simulink model "control_model_5"  (R2025b)
settings: Solver=VariableStepAuto  StartTime=0.0  StopTime=500  RelTol=1e-3
values from neighbouring files (symbols this model uses):
  Am = [0 1 0 0; -walpha^2 -2*zeta_alpha*walpha 0 0; 0 0 0 1; 0 0 -wgamma^2 -2*zeta_gamma*wgamma]    [main_v2.m]    (also in script_plane.m = [0 1; -wn^2 -2*zeta*wn])
  B = [0; Cm_delta*K/Iy; 0; 0]    [main_v2.m]    (also in script_plane.m = [0; Cm_delta/Iy])
  Bm = [0; walpha^2; 0; 0]    [main_v2.m]    (also in script_plane.m = [0; wn^2])
  c = 3.2    [main_v2.m]    (also in script_plane.m = 3.45)
  Cd0 = 0.02    [main_v2.m]
  Cl0 = 0.1    [main_v2.m]
  Cl_alpha = 5.7    [main_v2.m]
  Cm_0 = -0.8    [main_v2.m]
  Cm_delta = -0.5    [main_v2.m]    (also in script_plane.m = -1)
  Cm_q = -12    [main_v2.m]    (also in script_plane.m = -8)
  delta_max = deg2rad(25)    [main_v2.m]    (also in script_plane.m)
  desired_aoa = deg2rad(45)    [main_v2.m]    (also in script_plane.m = deg2rad(20))
  g = 9.81    [main_v2.m]
  gain_e = 0.1    [main_v2.m]    (also in script_plane.m = 50000)
  gain_r = 0.01    [main_v2.m]    (also in script_plane.m = 500000)
  gain_x = 0.00002    (= 2e-05)    [main_v2.m]    (also in script_plane.m = 500000)
  Iy = 160000    [main_v2.m]    (also in script_plane.m = 70000)
  K = 1/2 *rho * S *c    (= 58.8)    [main_v2.m]    (also in script_plane.m = 1908126.5175)
  k_d1 = 0.045    [main_v2.m]
  k_d2 = 0.08    [main_v2.m]
  kl = 3    [main_v2.m]
  Kr = 34.3*10^-3    (= 0.0343)    [main_v2.m]    (also in script_plane.m = -0.825)
  Kx = [19 -8 0 15]*10^-5    [main_v2.m]    (also in script_plane.m = [1.33 0.15])
  mass = 9000    [main_v2.m]    (also in script_plane.m = 12000)
  P = lyap(Am',Q)    [main_v2.m]    (also in script_plane.m)
  rate_of_change = 4    [main_v2.m]    (also in script_plane.m = 15)
  rate_of_freeze_angle = 1    [main_v2.m]
  rate_of_freeze_rate = 2    [main_v2.m]
  rho = 1.225    [main_v2.m]    (also in script_plane.m)
  S = 30    [main_v2.m]    (also in script_plane.m = 27.87)
  sigma_r = 0.001    [main_v2.m]    (also in script_plane.m = 0.0002)
  sigma_w = 0.001    [main_v2.m]    (also in script_plane.m = 0.0002)
  sigma_x = 0.001    [main_v2.m]    (also in script_plane.m = 0.0002)
  speed = 180    [main_v2.m]    (also in script_plane.m)
  thrust = 160000    [main_v2.m]
  W = [0 0 0 0 0]*10^-6    [main_v2.m]    (also in script_plane.m = [0 0 0 0])
  zeta_alpha = 1    [main_v2.m]
libraries: simulink_extras x22, simulink x2, slctrl_adaptive x1
settings Model: Creator=marti  LastModifiedBy=marti
settings SolverCC: ZeroCrossAlgorithm=Adaptive
settings DebuggingCC: MaskedZcDiagnostic=none  IgnoredZcDiagnostic=none

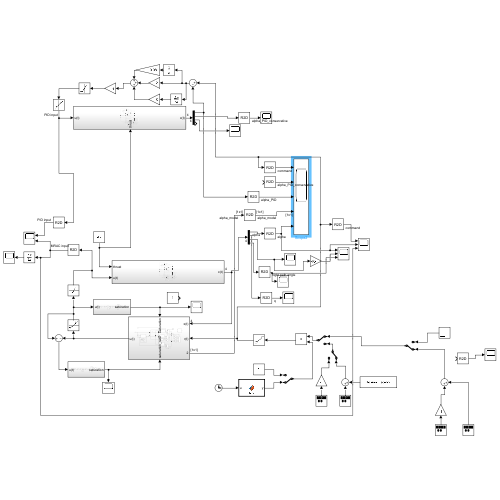
[thumbnail: Simulink's stored preview of the top-level diagram]
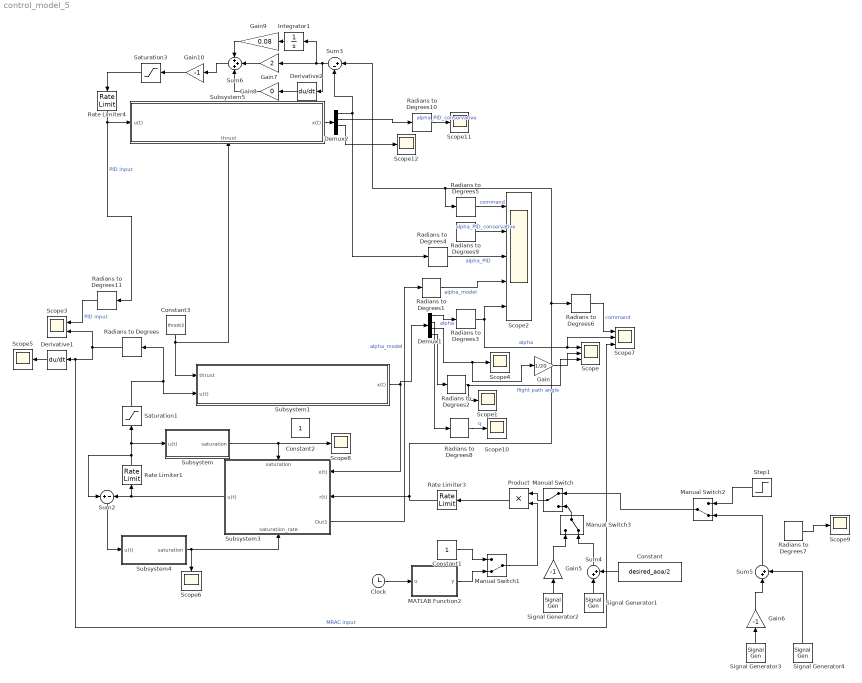
== system control_model_5 ==
  Clock : Clock
  Constant : Constant  Value=desired_aoa/2
  Constant1 : Constant
  Constant2 : Constant
  Constant3 : Constant  Value=thrust/3
  Demux1 : Demux
  Demux2 : Demux
  Derivative1 : Derivative
  Derivative2 : Derivative
  Gain : Gain  Gain=1/20
  Gain10 : Gain  Gain=-1
  Gain5 : Gain  Gain=-1
  Gain6 : Gain  Gain=-1
  Gain7 : Gain  Gain=2
  Gain8 : Gain  Gain=0
  Gain9 : Gain  Gain=0.08
  Integrator1 : Integrator
  MATLAB Function2 : MATLAB Function  TreatAsAtomicUnit=on
  Manual Switch : ManualSwitch
  Manual Switch1 : ManualSwitch  CurrentSetting=0
  Manual Switch2 : ManualSwitch  CurrentSetting=0
  Manual Switch3 : ManualSwitch  CurrentSetting=0
  Product : Product
  Radians to Degrees{,1..11} (12 alike) : simulink_extras/Transformations/Radians to Degrees
  Rate Limiter1 : RateLimiter  RisingSlewLimit=deg2rad(60)  FallingSlewLimit=-deg2rad(60)  SampleTimeMode=inherited
  Rate Limiter3 : RateLimiter  RisingSlewLimit=deg2rad(50)  FallingSlewLimit=-deg2rad(50)  SampleTimeMode=inherited
  Rate Limiter4 : RateLimiter  RisingSlewLimit=deg2rad(60)  FallingSlewLimit=-deg2rad(60)  SampleTimeMode=inherited
  Saturation1 : Saturate  UpperLimit=delta_max  LowerLimit=-delta_max  ZeroCross=off
  Saturation3 : Saturate  UpperLimit=delta_max  LowerLimit=-delta_max  ZeroCross=off
  Scope : Scope  NumInputPorts=3
      settings: ActiveDisplayYMinimum=-1  ActiveDisplayYMaximum=1  DataLoggingVariableName=ScopeData3
  Scope{1,4..6,8..12} (9 alike) : Scope
      Scope1 settings: ActiveDisplayYMinimum=-58.129213057968116  ActiveDisplayYMaximum=60.751359776371949  DataLoggingVariableName=ScopeData2
      Scope10 settings: ActiveDisplayYMinimum=-62.75251155469028  ActiveDisplayYMaximum=72.596643379359037  DataLoggingVariableName=ScopeData21
      Scope11 settings: ActiveDisplayYMinimum=-64.708088733273414  ActiveDisplayYMaximum=63.8671469407195  DataLoggingVariableName=ScopeData25
      Scope12 settings: ActiveDisplayYMinimum=129.65199773274497  ActiveDisplayYMaximum=311.01554736607403  DataLoggingVariableName=ScopeData26
      Scope4 settings: ActiveDisplayYMinimum=70.6671051217048  ActiveDisplayYMaximum=318.87721463336675  DataLoggingVariableName=ScopeData13
      Scope5 settings: ActiveDisplayYMinimum=-75.0023145799513  ActiveDisplayYMaximum=75.004597453327918  DataLoggingVariableName=ScopeData17
      Scope6 settings: ActiveDisplayYMinimum=-0.12499999999999997  ActiveDisplayYMaximum=1.125  DataLoggingVariableName=ScopeData12
      Scope8 settings: ActiveDisplayYMinimum=0.14902753825083676  ActiveDisplayYMaximum=1.0945524934597364  DataLoggingVariableName=ScopeData18
      Scope9 settings: ActiveDisplayYMinimum=-1  ActiveDisplayYMaximum=1  DataLoggingVariableName=ScopeData19
  Scope2 : Scope  NumInputPorts=5
      settings: ActiveDisplayYMinimum=-57.336392914968393  ActiveDisplayYMaximum=57.316790282004284  DataLoggingVariableName=ScopeData15
  Scope3 : Scope  NumInputPorts=2
      settings: ActiveDisplayYMinimum=-26.434953423968707  ActiveDisplayYMaximum=30.698276071875242  DataLoggingVariableName=ScopeData16
  Scope7 : Scope  NumInputPorts=3
      settings: ActiveDisplayYMinimum=-76.904040190876856  ActiveDisplayYMaximum=77.107808461045764  DataLoggingVariableName=ScopeData14
  Signal Generator1 : SignalGenerator  WaveForm=square  Amplitude=desired_aoa/2  Frequency=0.1  Units=rad/sec
  Signal Generator2 : SignalGenerator  WaveForm=square  Amplitude=desired_aoa  Frequency=0.2  Units=rad/sec
  Signal Generator3 : SignalGenerator  WaveForm=square  Amplitude=desired_aoa/2  Frequency=0.1  Units=rad/sec
  Signal Generator4 : SignalGenerator  WaveForm=square  Amplitude=desired_aoa/2  Frequency=0.05  Units=rad/sec
  Step1 : Step  Time=31.3  After=desired_aoa  SampleTime=0
  Subsystem : Subsystem
  Subsystem1 : Subsystem
  Subsystem3 : Subsystem
      settings: PortSchema="{\"entries\":[{\"content\":{\"sides\":[{\"content\":{\"connectorIds\":[\"Out2\",\"In1\",\"In2\"]},\"type\":\"ConnectorPlacement.EquallySpacedRectSide\",\"uuid\":\"2a5405b8-f474-466f-9064-f86b75893dd0\"},{\"content\":{\"connectorIds\":[\"Out1\"],\"side\":\"RIGHT\"},\"type\":\"ConnectorPlacement.EquallySpacedRectSide\",\"uuid\":\"ad673661-f4e9-494b-83cc-7452eec3fe31\"},{\"content\":{\"connectorIds\":[\"In3\"],\"side\":\"TOP\"},\"type\":\"ConnectorPlacement.EquallySpacedRectSide\",\"uuid\":\"21a76317-3288-4ff3-bd02-68708e86e3a8\"},{\"content\":{\"connectorIds\":[\"In4\"],\"side\":\"BOTTOM\"},\"type\":\"ConnectorPlacement.EquallySpacedRectSide\",\"uuid\":\"06318006-2373-43e5-8136-a784e8462fed\"}]},\"type\":\"ConnectorPlacement.EquallySpacedConnector\",\"uuid\":\"fc0ce599-928f-4c66-9629-0b98f2391e21\"}],\"packageUris\":[\"http://schema.mathworks.com/mf0/Connector/R2020b\"],\"version\":\"1.0\"}"
  Subsystem4 : Subsystem
  Subsystem5 : Subsystem
      settings: PortSchema="{\"entries\":[{\"content\":{\"sides\":[{\"content\":{\"connectorIds\":[\"In1\"]},\"type\":\"ConnectorPlacement.EquallySpacedRectSide\",\"uuid\":\"e785faf8-3185-4a85-a8dc-ea057f593b7d\"},{\"content\":{\"connectorIds\":[\"Out1\"],\"side\":\"RIGHT\"},\"type\":\"ConnectorPlacement.EquallySpacedRectSide\",\"uuid\":\"50c2acdd-3993-4760-8234-c723508cab38\"},{\"content\":{\"side\":\"TOP\"},\"type\":\"ConnectorPlacement.EquallySpacedRectSide\",\"uuid\":\"23fa212d-a38a-4506-9cd4-8e0f9463f517\"},{\"content\":{\"connectorIds\":[\"In2\"],\"side\":\"BOTTOM\"},\"type\":\"ConnectorPlacement.EquallySpacedRectSide\",\"uuid\":\"8bce308f-c5df-4db2-bea6-6d2a873f00b4\"}]},\"type\":\"ConnectorPlacement.EquallySpacedConnector\",\"uuid\":\"334871f8-06ef-498c-97e4-8f1bab52b431\"}],\"packageUris\":[\"http://schema.mathworks.com/mf0/Connector/R2020b\"],\"version\":\"1.0\"}"
  Sum2 : Sum  Inputs=+|-
  Sum3 : Sum  Inputs=|+-
  Sum4 : Sum  Inputs=|++
  Sum5 : Sum  Inputs=|++
  Sum6 : Sum  Inputs=+++
  wires:
  Radians to Degrees3/1 -> Scope7/2, Scope/1, Scope2/5  "alpha"
  Radians to Degrees4/1 -> Scope2/3  "alpha_PID"
  Signal Generator1/1 -> Sum4/1
  Derivative1/1 -> Scope5/1
  Subsystem3/1(u(t)) -> Sum2/2, Rate Limiter1/1
  Subsystem4/1(saturation) -> Subsystem3/3(saturation_rate), Scope6/1
  Subsystem3/2(Out1) -> Radians to Degrees1/1  "alpha_model"
  Saturation1/1 -> Radians to Degrees/1, Subsystem1/2(u(t))
  Radians to Degrees1/1 -> Scope2/4  "alpha_model"
  Constant/1 -> Sum4/2
  Manual Switch3/1 -> Manual Switch/2
  Sum2/1 -> Subsystem4/1(u(t))
  Radians to Degrees5/1 -> Scope2/1  "command"
  Radians to Degrees/1 -> Scope3/2, Scope7/3, Derivative1/1  "MRAC input"
  Sum4/1 -> Manual Switch3/2
  Demux1/3 -> Gain/1, Scope4/1
  Radians to Degrees2/1 -> Scope1/1, Scope/3  "flight path angle"
  Clock/1 -> MATLAB Function2/1(u)
  Manual Switch/1 -> Product/1
  Demux1/1 -> Radians to Degrees3/1  "alpha"
  Demux1/4 -> Radians to Degrees2/1
  Constant1/1 -> Manual Switch1/1
  MATLAB Function2/1(y) -> Manual Switch1/2
  Manual Switch1/1 -> Product/2
  Gain/1 -> Scope/2
  Subsystem/1(saturation) -> Scope8/1, Subsystem3/4(saturation)
  Rate Limiter1/1 -> Sum2/1, Saturation1/1, Subsystem/1(u(t))
  Signal Generator2/1 -> Gain5/1
  Gain5/1 -> Manual Switch3/1
  Radians to Degrees6/1 -> Scope7/1  "command"
  Subsystem1/1(x(t)) -> Demux1/1, Subsystem3/2(x(t))
  Constant3/1 -> Subsystem5/2(thrust), Subsystem1/1(thrust)
  Signal Generator3/1 -> Gain6/1
  Gain6/1 -> Sum5/1
  Signal Generator4/1 -> Sum5/2
  Radians to Degrees7/1 -> Scope9/1
  Radians to Degrees8/1 -> Scope10/1  "q"
  Demux1/2 -> Radians to Degrees8/1
  Subsystem5/1(x(t)) -> Demux2/1
  Gain8/1 -> Sum6/3
  Gain9/1 -> Sum6/1
  Sum3/1 -> Derivative2/1, Gain7/1, Integrator1/1
  Derivative2/1 -> Gain8/1
  Gain10/1 -> Saturation3/1
  Demux2/1 -> Radians to Degrees4/1, Sum3/2
  Rate Limiter4/1 -> Radians to Degrees11/1, Subsystem5/1(u(t))  "PID input"
  Sum6/1 -> Gain10/1
  Rate Limiter3/1 -> Subsystem3/1(r(t)), Radians to Degrees5/1, Sum3/1, Radians to Degrees6/1
  Saturation3/1 -> Rate Limiter4/1
  Gain7/1 -> Sum6/2
  Radians to Degrees9/1 -> Scope2/2  "alpha_PID_conservative"
  Integrator1/1 -> Gain9/1
  Demux2/2 -> Radians to Degrees10/1
  Radians to Degrees10/1 -> Scope11/1  "alpha_PID_conservative"
  Demux2/3 -> Scope12/1
  Radians to Degrees11/1 -> Scope3/1  "PID input"
  Product/1 -> Rate Limiter3/1
  Manual Switch2/1 -> Manual Switch/1
  Sum5/1 -> Manual Switch2/2
  Step1/1 -> Manual Switch2/1

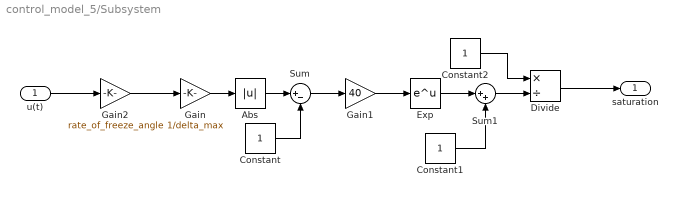
== system control_model_5/Subsystem ==
  u(t) : Inport
  Abs : Abs  SaturateOnIntegerOverflow=off
  Constant : Constant
  Constant1 : Constant
  Constant2 : Constant
  Divide : Product  Inputs=*/
  Exp : Math
  Gain : Gain  Gain=1/delta_max
  Gain1 : Gain  Gain=40
  Gain2 : Gain  Gain=rate_of_freeze_angle
  Sum : Sum  Inputs=|+-
  Sum1 : Sum  Inputs=|++
  saturation : Outport
  wires:
  Gain/1 -> Abs/1
  Abs/1 -> Sum/1
  Sum/1 -> Gain1/1
  Constant/1 -> Sum/2
  Gain1/1 -> Exp/1
  Exp/1 -> Sum1/1
  Constant1/1 -> Sum1/2
  Sum1/1 -> Divide/2
  Constant2/1 -> Divide/1
  Divide/1 -> saturation/1
  Gain2/1 -> Gain/1
  u(t)/1 -> Gain2/1

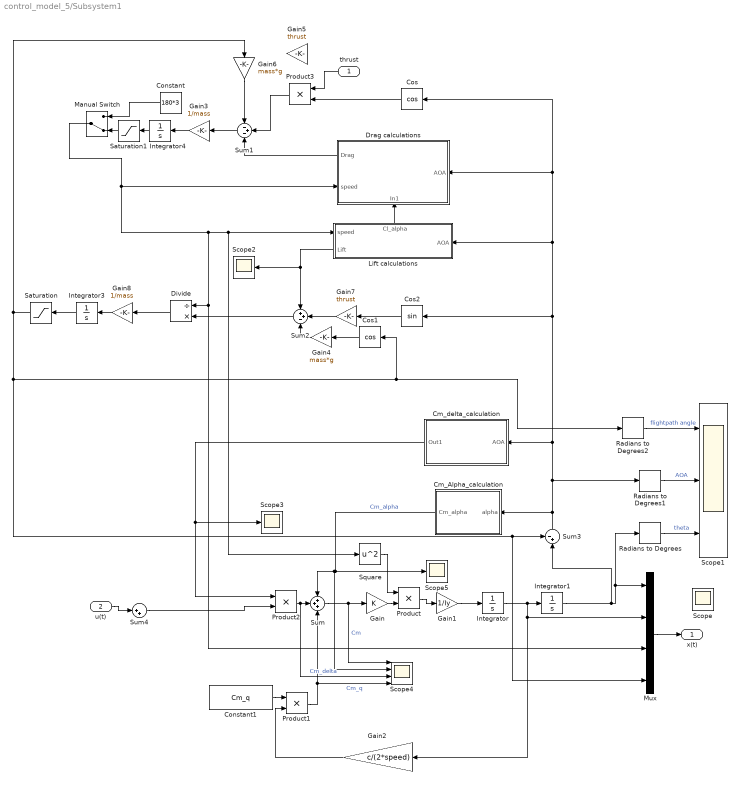
== system control_model_5/Subsystem1 ==
  thrust : Inport
  u(t) : Inport  Port=2
  Cm_Alpha_calculation : Subsystem
  Cm_delta_calculation : Subsystem
  Constant : Constant  Value=180*3
  Constant1 : Constant  Value=Cm_q
  Cos : Trigonometry  Operator=cos
  Cos1 : Trigonometry  Operator=cos
  Cos2 : Trigonometry
  Divide : Product  Inputs=/*
  Drag calculations : Subsystem
      settings: PortSchema="{\"entries\":[{\"content\":{\"sides\":[{\"content\":{\"connectorIds\":[\"Out1\",\"In1\"]},\"type\":\"ConnectorPlacement.EquallySpacedRectSide\",\"uuid\":\"d271dd9c-4b6b-493d-a484-ea343b2a7ea5\"},{\"content\":{\"connectorIds\":[\"In3\"],\"side\":\"RIGHT\"},\"type\":\"ConnectorPlacement.EquallySpacedRectSide\",\"uuid\":\"1c3a3b91-ae49-4f86-b72d-44481f1c47ea\"},{\"content\":{\"side\":\"TOP\"},\"type\":\"ConnectorPlacement.EquallySpacedRectSide\",\"uuid\":\"ad2c4e7a-6e16-439a-a8ce-91c789fc2dda\"},{\"content\":{\"connectorIds\":[\"In2\"],\"side\":\"BOTTOM\"},\"type\":\"ConnectorPlacement.EquallySpacedRectSide\",\"uuid\":\"1d27e3d2-8ebb-4b91-86b1-b9e0cbaba979\"}]},\"type\":\"ConnectorPlacement.EquallySpacedConnector\",\"uuid\":\"312dc24d-03ba-4f6d-95f4-f718ce8b3ee8\"}],\"packageUris\":[\"http://schema.mathworks.com/mf0/Connector/R2020b\"],\"version\":\"1.0\"}"
  Gain : Gain  Gain=K
  Gain1 : Gain  Gain=1/Iy
  Gain2 : Gain  Gain=c/(2*speed)
  Gain3 : Gain  Gain=1/mass
  Gain4 : Gain  Gain=mass*g
  Gain5 : Gain  Gain=thrust
  Gain6 : Gain  Gain=mass*g
  Gain7 : Gain  Gain=thrust
  Gain8 : Gain  Gain=1/mass
  Integrator : Integrator
  Integrator1 : Integrator
  Integrator3 : Integrator
  Integrator4 : Integrator  InitialCondition=speed
  Lift calculations : Subsystem
      settings: PortSchema="{\"entries\":[{\"content\":{\"sides\":[{\"content\":{\"connectorIds\":[\"In1\",\"Out2\"]},\"type\":\"ConnectorPlacement.EquallySpacedRectSide\",\"uuid\":\"5246f013-813c-4805-903b-98ed221a01a8\"},{\"content\":{\"connectorIds\":[\"In2\"],\"side\":\"RIGHT\"},\"type\":\"ConnectorPlacement.EquallySpacedRectSide\",\"uuid\":\"452079bc-9591-4c95-a88f-c45e08717f6a\"},{\"content\":{\"connectorIds\":[\"Out1\"],\"side\":\"TOP\"},\"type\":\"ConnectorPlacement.EquallySpacedRectSide\",\"uuid\":\"f365ba97-25c1-460b-8c6b-56706c8bd897\"}]},\"type\":\"ConnectorPlacement.EquallySpacedConnector\",\"uuid\":\"7294dbab-9b96-4a0b-a23a-2bd2309fe32e\"}],\"packageUris\":[\"http://schema.mathworks.com/mf0/Connector/R2020b\"],\"version\":\"1.0\"}"
  Manual Switch : ManualSwitch  CurrentSetting=0
  Mux : Mux
  Product{,1..3} (4 alike) : Product
  Radians to Degrees : simulink_extras/Transformations/Radians to Degrees
  Radians to Degrees1 : simulink_extras/Transformations/Radians to Degrees
  Radians to Degrees2 : simulink_extras/Transformations/Radians to Degrees
  Saturation : Saturate  UpperLimit=deg2rad(90)  LowerLimit=-deg2rad(90)
  Saturation1 : Saturate  UpperLimit=1000  LowerLimit=0
  Scope{,2..3,5} (4 alike) : Scope
      Scope settings: ActiveDisplayYMinimum=-0.01377254423088568  ActiveDisplayYMaximum=0.024994154646199356
      Scope2 settings: ActiveDisplayYMinimum=52037.469544787207  ActiveDisplayYMaximum=126455.77992982147  DataLoggingVariableName=ScopeData5
      Scope3 settings: ActiveDisplayYMinimum=-1  ActiveDisplayYMaximum=1  DataLoggingVariableName=ScopeData4
      Scope5 settings: ActiveDisplayYMinimum=-1  ActiveDisplayYMaximum=1  DataLoggingVariableName=ScopeData10
  Scope1 : Scope  NumInputPorts=3
      settings: ActiveDisplayYMinimum=-22.932754420489626  ActiveDisplayYMaximum=15.066132831552849
  Scope4 : Scope  NumInputPorts=4
      settings: ActiveDisplayYMinimum=-1  ActiveDisplayYMaximum=1  DataLoggingVariableName=ScopeData24
  Square : Math  Operator=square
  Sum : Sum  Inputs=+++
  Sum1 : Sum  Inputs=-+-
  Sum2 : Sum  Inputs=++-
  Sum3 : Sum  Inputs=-+|
  Sum4 : Sum  Inputs=|++
  x(t) : Outport
  wires:
  Product2/1 -> Scope4/3, Sum/2  "Cm_delta"
  Gain1/1 -> Integrator/1
  Integrator/1 -> Mux/2, Gain2/1, Integrator1/1
  Constant1/1 -> Product1/1
  Product1/1 -> Scope4/4, Sum/3  "Cm_q"
  Gain2/1 -> Product1/2
  Integrator1/1 -> Sum3/2, Mux/1, Radians to Degrees/1
  Cm_Alpha_calculation/1(Cm_alpha) -> Scope4/2, Sum/1, Scope5/1  "Cm_alpha"
  Cm_delta_calculation/1(Out1) -> Product2/1, Scope3/1
  Lift calculations/2(Lift) -> Sum2/1, Scope2/1
  Lift calculations/1(Cl_alpha) -> Drag calculations/2(In1)
  Drag calculations/1(Drag) -> Sum1/3
  Sum1/1 -> Gain3/1
  Cos1/1 -> Gain4/1
  Gain6/1 -> Sum1/1
  Gain4/1 -> Sum2/3
  Gain7/1 -> Sum2/2
  Cos2/1 -> Gain7/1
  Sum2/1 -> Divide/2
  Divide/1 -> Gain8/1
  Gain8/1 -> Integrator3/1
  Sum3/1 -> Radians to Degrees1/1, Cos2/1, Cos/1, Drag calculations/3(AOA), Lift calculations/2(AOA), Cm_delta_calculation/1(AOA), Cm_Alpha_calculation/1(alpha)
  Gain/1 -> Product/2
  Product/1 -> Gain1/1
  Square/1 -> Product/1
  Radians to Degrees/1 -> Scope1/3  "theta"
  Radians to Degrees1/1 -> Scope1/2  "AOA"
  Radians to Degrees2/1 -> Scope1/1  "flightpath angle"
  Integrator3/1 -> Saturation/1
  Saturation/1 -> Mux/4, Sum3/1, Cos1/1, Radians to Degrees2/1, Gain6/1
  Mux/1 -> x(t)/1
  u(t)/1 -> Sum4/1
  Sum4/1 -> Product2/2
  Manual Switch/1 -> Mux/3, Divide/1, Square/1, Lift calculations/1(speed), Drag calculations/1(speed)
  Cos/1 -> Product3/2
  Product3/1 -> Sum1/2
  thrust/1 -> Product3/1
  Sum/1 -> Scope4/1, Gain/1  "Cm"
  Gain3/1 -> Integrator4/1
  Constant/1 -> Manual Switch/1
  Saturation1/1 -> Manual Switch/2
  Integrator4/1 -> Saturation1/1

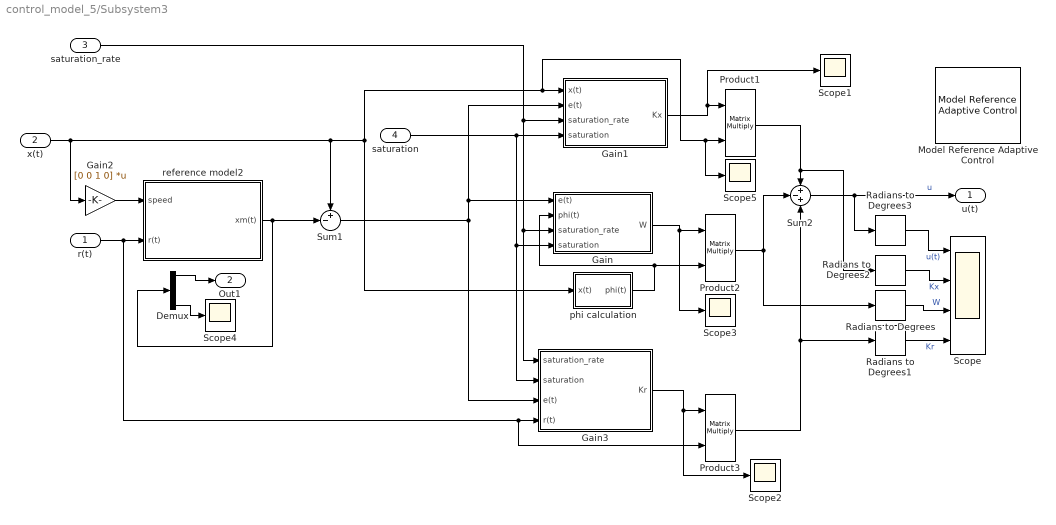
== system control_model_5/Subsystem3 ==
  r(t) : Inport
  x(t) : Inport  Port=2
  saturation_rate : Inport  Port=3
  saturation : Inport  Port=4
  Demux : Demux
  Gain : Subsystem
  Gain1 : Subsystem
  Gain2 : Gain  Gain=[0 0 1 0]  Multiplication=Matrix(K*u) (u vector)
  Gain3 : Subsystem
  Model Reference Adaptive Control : slctrl_adaptive/Model Reference Adaptive Control  selectType=Direct  A=0  B=1  Ahat=0  ALrEnable=on  gamma_a=1  ALrEnableMod=on  Bhat=1  BLrEnable=on  gamma_b=1  BLrEnableMod=on  externalKtauEnable=off  k_tau=-1  estParamOutput=off  Am=-1  Bm=1  kx=0  FBLrEnable=on  gamma_kx=1  FBLrEnableMod=on  kr=0  FFLrEnable=on  gamma_kr=1  FFLrEnableMod=on  AdaptEnable=on  gamma=1  WLrEnableMod=on  Q=1  FeatureTypeOptions=State  shlHiddenLayerSize=10  gamma_V=0.1  nCen=20  cSpanMin=-1  cSpanMax=1  cSig=5  adaptiveCntrlOutport=off  modChoice=None  sigma_val=0.1  DiscreteEnable=off  Ts=0.05  IntegrationMethods=Forward Euler
      settings: LibrarySourceBlock=slctrlblks/Adaptive Control/Model Reference Adaptive Control
  Product1 : Product  Multiplication=Matrix(*)
  Product2 : Product  Multiplication=Matrix(*)
  Product3 : Product  Multiplication=Matrix(*)
  Radians to Degrees{,1..3} (4 alike) : simulink_extras/Transformations/Radians to Degrees
  Scope : Scope  NumInputPorts=4
      settings: ActiveDisplayYMinimum=-28.663135806268023  ActiveDisplayYMaximum=27.287900279681331  DataLoggingVariableName=ScopeData6
  Scope{1..5} (5 alike) : Scope
      Scope1 settings: ActiveDisplayYMinimum=-0.00011374999999999999  ActiveDisplayYMaximum=0.00022375  DataLoggingVariableName=ScopeData7
      Scope2 settings: ActiveDisplayYMinimum=-0.00029861573834764031  ActiveDisplayYMaximum=0.0024448482326404589  DataLoggingVariableName=ScopeData8
      Scope3 settings: ActiveDisplayYMinimum=-1.1448700726841352E-8  ActiveDisplayYMaximum=5.6474676960149013E-9  DataLoggingVariableName=ScopeData9
      Scope4 settings: ActiveDisplayYMinimum=-74.409916279159262  ActiveDisplayYMaximum=8.26776916563939  DataLoggingVariableName=ScopeData20
      Scope5 settings: ActiveDisplayYMinimum=-79.2606396623334  ActiveDisplayYMaximum=704.98996940397183  DataLoggingVariableName=ScopeData22
  Sum1 : Sum  Inputs=+-|
  Sum2 : Sum  Inputs=+-+
  phi calculation : Subsystem
  reference model2 : Subsystem  TreatAsAtomicUnit=on
  u(t) : Outport
  Out1 : Outport  Port=2
  wires:
  r(t)/1 -> Product3/2, Gain3/4(r(t)), reference model2/2(r(t))
  reference model2/1(xm(t)) -> Sum1/2, Demux/1
  x(t)/1 -> Gain1/1(x(t)), Scope5/1, Product1/2, phi calculation/1(x(t)), Sum1/1, Gain2/1
  Product1/1 -> Radians to Degrees2/1, Sum2/1
  Gain/1(W) -> Scope3/1, Product2/1
  Gain1/1(Kx) -> Scope1/1, Product1/1
  Gain3/1(Kr) -> Scope2/1, Product3/1
  Product3/1 -> Sum2/3, Radians to Degrees1/1
  Product2/1 -> Radians to Degrees/1, Sum2/2
  Radians to Degrees2/1 -> Scope/2  "Kx"
  Radians to Degrees/1 -> Scope/3  "W"
  Radians to Degrees1/1 -> Scope/4  "Kr"
  Sum2/1 -> Radians to Degrees3/1, u(t)/1  "u"
  Radians to Degrees3/1 -> Scope/1  "u(t)"
  saturation_rate/1 -> Gain1/3(saturation_rate), Gain3/1(saturation_rate), Gain/3(saturation_rate)
  saturation/1 -> Gain3/2(saturation), Gain/4(saturation), Gain1/4(saturation)
  phi calculation/1(phi(t)) -> Gain/2(phi(t)), Product2/2
  Demux/1 -> Out1/1
  Demux/4 -> Scope4/1
  Gain2/1 -> reference model2/1(speed)
  Sum1/1 -> Gain3/3(e(t)), Gain/1(e(t)), Gain1/2(e(t))

== system control_model_5/Subsystem4 ==
  u(t) : Inport
  Abs : Abs  SaturateOnIntegerOverflow=off
  Constant : Constant
  Constant1 : Constant
  Constant2 : Constant
  Divide : Product  Inputs=*/
  Exp : Math
  Gain : Gain  Gain=1/delta_max
  Gain1 : Gain  Gain=40
  Gain2 : Gain  Gain=rate_of_freeze_rate
  Sum : Sum  Inputs=|+-
  Sum1 : Sum  Inputs=|++
  saturation : Outport
  wires:
  Gain/1 -> Abs/1
  Abs/1 -> Sum/1
  Sum/1 -> Gain1/1
  Constant/1 -> Sum/2
  Gain1/1 -> Exp/1
  Exp/1 -> Sum1/1
  Constant1/1 -> Sum1/2
  Sum1/1 -> Divide/2
  Constant2/1 -> Divide/1
  Divide/1 -> saturation/1
  Gain2/1 -> Gain/1
  u(t)/1 -> Gain2/1

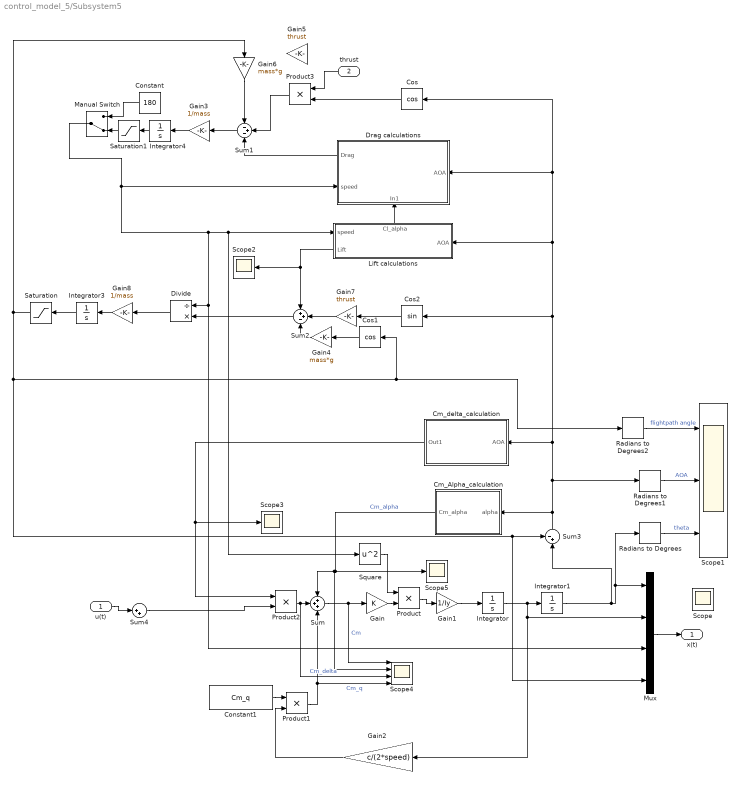
== system control_model_5/Subsystem5 ==
  u(t) : Inport
  thrust : Inport  Port=2
  Cm_Alpha_calculation : Subsystem
  Cm_delta_calculation : Subsystem
  Constant : Constant  Value=180
  Constant1 : Constant  Value=Cm_q
  Cos : Trigonometry  Operator=cos
  Cos1 : Trigonometry  Operator=cos
  Cos2 : Trigonometry
  Divide : Product  Inputs=/*
  Drag calculations : Subsystem
      settings: PortSchema="{\"entries\":[{\"content\":{\"sides\":[{\"content\":{\"connectorIds\":[\"Out1\",\"In1\"]},\"type\":\"ConnectorPlacement.EquallySpacedRectSide\",\"uuid\":\"d271dd9c-4b6b-493d-a484-ea343b2a7ea5\"},{\"content\":{\"connectorIds\":[\"In3\"],\"side\":\"RIGHT\"},\"type\":\"ConnectorPlacement.EquallySpacedRectSide\",\"uuid\":\"1c3a3b91-ae49-4f86-b72d-44481f1c47ea\"},{\"content\":{\"side\":\"TOP\"},\"type\":\"ConnectorPlacement.EquallySpacedRectSide\",\"uuid\":\"ad2c4e7a-6e16-439a-a8ce-91c789fc2dda\"},{\"content\":{\"connectorIds\":[\"In2\"],\"side\":\"BOTTOM\"},\"type\":\"ConnectorPlacement.EquallySpacedRectSide\",\"uuid\":\"1d27e3d2-8ebb-4b91-86b1-b9e0cbaba979\"}]},\"type\":\"ConnectorPlacement.EquallySpacedConnector\",\"uuid\":\"312dc24d-03ba-4f6d-95f4-f718ce8b3ee8\"}],\"packageUris\":[\"http://schema.mathworks.com/mf0/Connector/R2020b\"],\"version\":\"1.0\"}"
  Gain : Gain  Gain=K
  Gain1 : Gain  Gain=1/Iy
  Gain2 : Gain  Gain=c/(2*speed)
  Gain3 : Gain  Gain=1/mass
  Gain4 : Gain  Gain=mass*g
  Gain5 : Gain  Gain=thrust
  Gain6 : Gain  Gain=mass*g
  Gain7 : Gain  Gain=thrust
  Gain8 : Gain  Gain=1/mass
  Integrator : Integrator
  Integrator1 : Integrator
  Integrator3 : Integrator
  Integrator4 : Integrator  InitialCondition=speed
  Lift calculations : Subsystem
      settings: PortSchema="{\"entries\":[{\"content\":{\"sides\":[{\"content\":{\"connectorIds\":[\"In1\",\"Out2\"]},\"type\":\"ConnectorPlacement.EquallySpacedRectSide\",\"uuid\":\"5246f013-813c-4805-903b-98ed221a01a8\"},{\"content\":{\"connectorIds\":[\"In2\"],\"side\":\"RIGHT\"},\"type\":\"ConnectorPlacement.EquallySpacedRectSide\",\"uuid\":\"452079bc-9591-4c95-a88f-c45e08717f6a\"},{\"content\":{\"connectorIds\":[\"Out1\"],\"side\":\"TOP\"},\"type\":\"ConnectorPlacement.EquallySpacedRectSide\",\"uuid\":\"f365ba97-25c1-460b-8c6b-56706c8bd897\"}]},\"type\":\"ConnectorPlacement.EquallySpacedConnector\",\"uuid\":\"7294dbab-9b96-4a0b-a23a-2bd2309fe32e\"}],\"packageUris\":[\"http://schema.mathworks.com/mf0/Connector/R2020b\"],\"version\":\"1.0\"}"
  Manual Switch : ManualSwitch  CurrentSetting=0
  Mux : Mux
  Product{,1..3} (4 alike) : Product
  Radians to Degrees : simulink_extras/Transformations/Radians to Degrees
  Radians to Degrees1 : simulink_extras/Transformations/Radians to Degrees
  Radians to Degrees2 : simulink_extras/Transformations/Radians to Degrees
  Saturation : Saturate  UpperLimit=deg2rad(90)  LowerLimit=-deg2rad(90)
  Saturation1 : Saturate  UpperLimit=1000  LowerLimit=0
  Scope{,2..3,5} (4 alike) : Scope
      Scope settings: ActiveDisplayYMinimum=-0.01377254423088568  ActiveDisplayYMaximum=0.024994154646199356
      Scope2 settings: ActiveDisplayYMinimum=52037.469544787207  ActiveDisplayYMaximum=126455.77992982147  DataLoggingVariableName=ScopeData5
      Scope3 settings: ActiveDisplayYMinimum=-1  ActiveDisplayYMaximum=1  DataLoggingVariableName=ScopeData4
      Scope5 settings: ActiveDisplayYMinimum=-1  ActiveDisplayYMaximum=1  DataLoggingVariableName=ScopeData10
  Scope1 : Scope  NumInputPorts=3
      settings: ActiveDisplayYMinimum=-22.932754420489626  ActiveDisplayYMaximum=15.066132831552849
  Scope4 : Scope  NumInputPorts=4
      settings: ActiveDisplayYMinimum=-1  ActiveDisplayYMaximum=1  DataLoggingVariableName=ScopeData24
  Square : Math  Operator=square
  Sum : Sum  Inputs=+++
  Sum1 : Sum  Inputs=-+-
  Sum2 : Sum  Inputs=++-
  Sum3 : Sum  Inputs=-+|
  Sum4 : Sum  Inputs=|++
  x(t) : Outport
  wires:
  Product2/1 -> Scope4/3, Sum/2  "Cm_delta"
  Gain1/1 -> Integrator/1
  Integrator/1 -> Mux/2, Gain2/1, Integrator1/1
  Constant1/1 -> Product1/1
  Product1/1 -> Scope4/4, Sum/3  "Cm_q"
  Gain2/1 -> Product1/2
  Integrator1/1 -> Sum3/2, Mux/1, Radians to Degrees/1
  Cm_Alpha_calculation/1(Cm_alpha) -> Scope4/2, Sum/1, Scope5/1  "Cm_alpha"
  Cm_delta_calculation/1(Out1) -> Product2/1, Scope3/1
  Lift calculations/2(Lift) -> Sum2/1, Scope2/1
  Lift calculations/1(Cl_alpha) -> Drag calculations/2(In1)
  Drag calculations/1(Drag) -> Sum1/3
  Sum1/1 -> Gain3/1
  Cos1/1 -> Gain4/1
  Gain6/1 -> Sum1/1
  Gain4/1 -> Sum2/3
  Gain7/1 -> Sum2/2
  Cos2/1 -> Gain7/1
  Sum2/1 -> Divide/2
  Divide/1 -> Gain8/1
  Gain8/1 -> Integrator3/1
  Sum3/1 -> Radians to Degrees1/1, Cos2/1, Cos/1, Drag calculations/3(AOA), Lift calculations/2(AOA), Cm_delta_calculation/1(AOA), Cm_Alpha_calculation/1(alpha)
  Gain/1 -> Product/2
  Product/1 -> Gain1/1
  Square/1 -> Product/1
  Radians to Degrees/1 -> Scope1/3  "theta"
  Radians to Degrees1/1 -> Scope1/2  "AOA"
  Radians to Degrees2/1 -> Scope1/1  "flightpath angle"
  Integrator3/1 -> Saturation/1
  Saturation/1 -> Mux/4, Sum3/1, Cos1/1, Radians to Degrees2/1, Gain6/1
  Mux/1 -> x(t)/1
  u(t)/1 -> Sum4/1
  Sum4/1 -> Product2/2
  Manual Switch/1 -> Mux/3, Divide/1, Square/1, Lift calculations/1(speed), Drag calculations/1(speed)
  Cos/1 -> Product3/2
  Product3/1 -> Sum1/2
  thrust/1 -> Product3/1
  Sum/1 -> Scope4/1, Gain/1  "Cm"
  Gain3/1 -> Integrator4/1
  Constant/1 -> Manual Switch/1
  Saturation1/1 -> Manual Switch/2
  Integrator4/1 -> Saturation1/1

== system control_model_5/Subsystem1/Cm_Alpha_calculation ==
  alpha : Inport
  Constant : Constant
  Constant1 : Constant
  Divide : Product  Inputs=*/
  Gain : Gain  Gain=1/deg2rad(15)
  Gain7 : Gain  Gain=Cm_0
  Product : Product
  Scope5 : Scope
      settings: ActiveDisplayYMinimum=-1  ActiveDisplayYMaximum=1  DataLoggingVariableName=ScopeData11
  Square : Math  Operator=square
  Sum : Sum  Inputs=|++
  Cm_alpha : Outport
  wires:
  Product/1 -> Cm_alpha/1
  Gain7/1 -> Scope5/1, Product/2
  Gain/1 -> Square/1
  alpha/1 -> Gain/1, Product/1
  Square/1 -> Sum/1
  Constant/1 -> Sum/2
  Sum/1 -> Divide/2
  Divide/1 -> Gain7/1
  Constant1/1 -> Divide/1

== system control_model_5/Subsystem1/Cm_delta_calculation ==
  AOA : Inport
  Constant11 : Constant  Value=Cm_delta
  Constant2 : Constant
  Divide : Product  Inputs=/*
  Gain5 : Gain  Gain=rate_of_change
  Square : Math  Operator=square
  Sum4 : Sum  Inputs=++|
  Out1 : Outport
  wires:
  Gain5/1 -> Sum4/2
  Constant2/1 -> Sum4/1
  Divide/1 -> Out1/1
  Sum4/1 -> Divide/1
  Constant11/1 -> Divide/2
  Square/1 -> Gain5/1
  AOA/1 -> Square/1

== system control_model_5/Subsystem1/Drag calculations ==
  speed : Inport
  In1 : Inport  Port=2
  AOA : Inport  Port=3
  Constant3 : Constant  Value=Cd0
  Gain5 : Gain  Gain=k_d2
  Gain6 : Gain  Gain=k_d1
  Gain7 : Gain  Gain=S*1/2*rho
  Product : Product
  Square : Math  Operator=square
  Square1 : Math  Operator=square
  Square2 : Math  Operator=square
  Sum3 : Sum  Inputs=+++
  Drag : Outport
  wires:
  Square1/1 -> Gain6/1
  Square2/1 -> Gain5/1
  Product/1 -> Drag/1
  Sum3/1 -> Gain7/1
  Gain6/1 -> Sum3/3
  Gain7/1 -> Product/2
  Constant3/1 -> Sum3/1
  Square/1 -> Product/1
  Gain5/1 -> Sum3/2
  AOA/1 -> Square2/1
  In1/1 -> Square1/1
  speed/1 -> Square/1

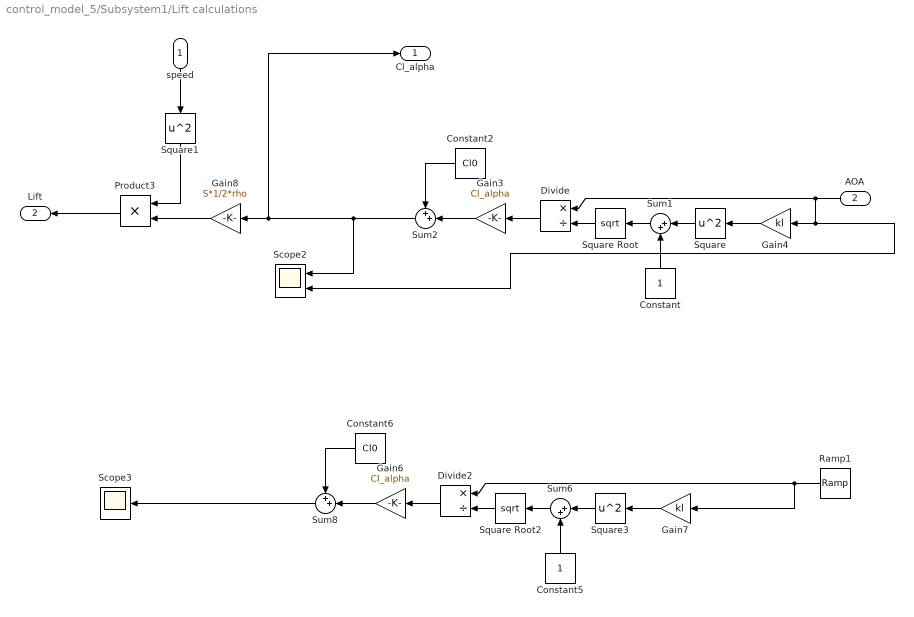
== system control_model_5/Subsystem1/Lift calculations ==
  speed : Inport
  AOA : Inport  Port=2
  Constant : Constant
  Constant2 : Constant  Value=Cl0
  Constant5 : Constant
  Constant6 : Constant  Value=Cl0
  Divide : Product  Inputs=*/
  Divide2 : Product  Inputs=*/
  Gain3 : Gain  Gain=Cl_alpha
  Gain4 : Gain  Gain=kl
  Gain6 : Gain  Gain=Cl_alpha
  Gain7 : Gain  Gain=kl
  Gain8 : Gain  Gain=S*1/2*rho
  Product3 : Product
  Ramp1 : simulink/Sources/Ramp  slope=deg2rad(1)  start=0  InitialOutput=-deg2rad(60)
  Scope2 : Scope  NumInputPorts=2
      settings: ActiveDisplayYMinimum=-3.0358993033761661  ActiveDisplayYMaximum=1.5205805122741798  DataLoggingVariableName=ScopeData9
  Scope3 : Scope
      settings: ActiveDisplayYMinimum=-2.1631149707231323  ActiveDisplayYMaximum=2.3631149707231325  DataLoggingVariableName=ScopeData23
  Square : Math  Operator=square
  Square Root : Sqrt
  Square Root2 : Sqrt
  Square1 : Math  Operator=square
  Square3 : Math  Operator=square
  Sum1 : Sum  Inputs=|++
  Sum2 : Sum  Inputs=++|
  Sum6 : Sum  Inputs=|++
  Sum8 : Sum  Inputs=++|
  Cl_alpha : Outport
  Lift : Outport  Port=2
  wires:
  Square/1 -> Sum1/1
  Square Root/1 -> Divide/2
  Gain3/1 -> Sum2/2
  Constant2/1 -> Sum2/1
  AOA/1 -> Divide/1, Scope2/2, Gain4/1
  Gain4/1 -> Square/1
  Gain8/1 -> Product3/2
  Constant/1 -> Sum1/2
  Divide/1 -> Gain3/1
  Product3/1 -> Lift/1
  Sum1/1 -> Square Root/1
  Square1/1 -> Product3/1
  speed/1 -> Square1/1
  Sum2/1 -> Cl_alpha/1, Gain8/1, Scope2/1
  Square3/1 -> Sum6/1
  Ramp1/1 -> Divide2/1, Gain7/1
  Gain7/1 -> Square3/1
  Gain6/1 -> Sum8/2
  Sum6/1 -> Square Root2/1
  Divide2/1 -> Gain6/1
  Constant6/1 -> Sum8/1
  Constant5/1 -> Sum6/2
  Square Root2/1 -> Divide2/2
  Sum8/1 -> Scope3/1

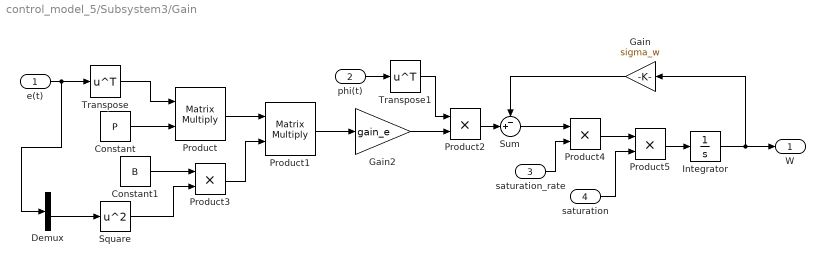
== system control_model_5/Subsystem3/Gain ==
  e(t) : Inport
  phi(t) : Inport  Port=2
  saturation_rate : Inport  Port=3
  saturation : Inport  Port=4
  Constant : Constant  Value=P  VectorParams1D=off
  Constant1 : Constant  Value=B  VectorParams1D=off
  Demux : Demux
  Gain : Gain  Gain=sigma_w
  Gain2 : Gain  Gain=gain_e
  Integrator : Integrator  InitialCondition=W
  Product : Product  Multiplication=Matrix(*)
  Product1 : Product  Multiplication=Matrix(*)
  Product{2..5} (4 alike) : Product
  Square : Math  Operator=square
  Sum : Sum  Inputs=-+|
  Transpose : Math  Operator=transpose
  Transpose1 : Math  Operator=transpose
  W : Outport
  wires:
  Product1/1 -> Gain2/1
  Product/1 -> Product1/1
  Gain2/1 -> Product2/2
  Constant/1 -> Product/2
  Transpose/1 -> Product/1
  Integrator/1 -> W/1, Gain/1
  phi(t)/1 -> Transpose1/1
  Transpose1/1 -> Product2/1
  Product2/1 -> Sum/2
  Gain/1 -> Sum/1
  saturation/1 -> Product5/2
  saturation_rate/1 -> Product4/2
  Sum/1 -> Product4/1
  Product4/1 -> Product5/1
  Product5/1 -> Integrator/1
  Demux/3 -> Square/1
  e(t)/1 -> Demux/1, Transpose/1
  Square/1 -> Product3/2
  Constant1/1 -> Product3/1
  Product3/1 -> Product1/2

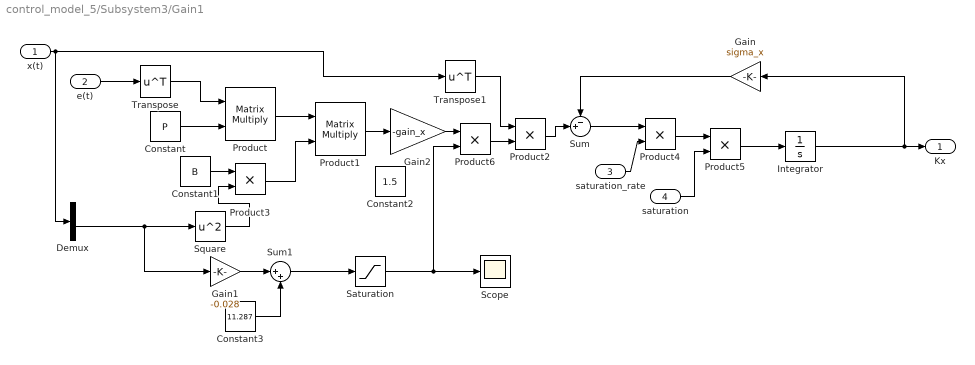
== system control_model_5/Subsystem3/Gain1 ==
  x(t) : Inport
  e(t) : Inport  Port=2
  saturation_rate : Inport  Port=3
  saturation : Inport  Port=4
  Constant : Constant  Value=P  VectorParams1D=off
  Constant1 : Constant  Value=B  VectorParams1D=off
  Constant2 : Constant  Value=1.5
  Constant3 : Constant  Value=11.287
  Demux : Demux
  Gain : Gain  Gain=sigma_x
  Gain1 : Gain  Gain=-0.028
  Gain2 : Gain  Gain=-gain_x
  Integrator : Integrator  InitialCondition=Kx
  Product : Product  Multiplication=Matrix(*)
  Product1 : Product  Multiplication=Matrix(*)
  Product{2..6} (5 alike) : Product
  Saturation : Saturate  UpperLimit=4.5  LowerLimit=1
  Scope : Scope
      settings: ActiveDisplayYMinimum=-1  ActiveDisplayYMaximum=1  DataLoggingVariableName=ScopeData28
  Square : Math  Operator=square
  Sum : Sum  Inputs=-+|
  Sum1 : Sum  Inputs=|++
  Transpose : Math  Operator=transpose
  Transpose1 : Math  Operator=transpose
  Kx : Outport
  wires:
  Product1/1 -> Gain2/1
  Product/1 -> Product1/1
  e(t)/1 -> Transpose/1
  Constant/1 -> Product/2
  Transpose/1 -> Product/1
  x(t)/1 -> Transpose1/1, Demux/1
  Transpose1/1 -> Product2/1
  Product2/1 -> Sum/2
  Gain/1 -> Sum/1
  Sum/1 -> Product4/1
  Product4/1 -> Product5/1
  Product5/1 -> Integrator/1
  saturation_rate/1 -> Product4/2
  saturation/1 -> Product5/2
  Constant1/1 -> Product3/1
  Product3/1 -> Product1/2
  Demux/3 -> Gain1/1, Square/1
  Integrator/1 -> Kx/1, Gain/1
  Gain2/1 -> Product6/1
  Product6/1 -> Product2/2
  Square/1 -> Product3/2
  Gain1/1 -> Sum1/1
  Constant3/1 -> Sum1/2
  Sum1/1 -> Saturation/1
  Saturation/1 -> Scope/1, Product6/2

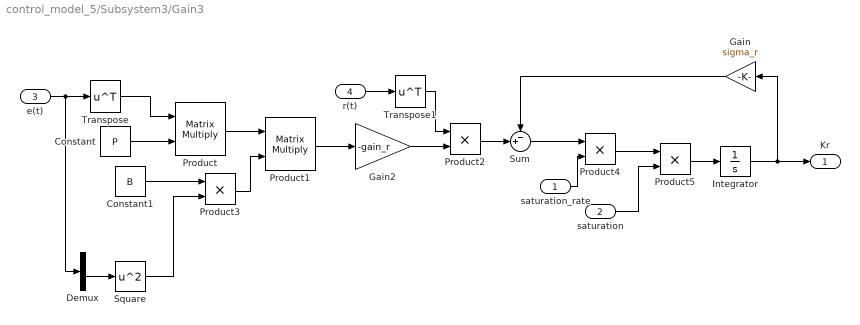
== system control_model_5/Subsystem3/Gain3 ==
  saturation_rate : Inport
  saturation : Inport  Port=2
  e(t) : Inport  Port=3
  r(t) : Inport  Port=4
  Constant : Constant  Value=P  VectorParams1D=off
  Constant1 : Constant  Value=B  VectorParams1D=off
  Demux : Demux
  Gain : Gain  Gain=sigma_r
  Gain2 : Gain  Gain=-gain_r
  Integrator : Integrator  InitialCondition=Kr
  Product : Product  Multiplication=Matrix(*)
  Product1 : Product  Multiplication=Matrix(*)
  Product{2..5} (4 alike) : Product
  Square : Math  Operator=square
  Sum : Sum  Inputs=-+|
  Transpose : Math  Operator=transpose
  Transpose1 : Math  Operator=transpose
  Kr : Outport
  wires:
  Product1/1 -> Gain2/1
  Product/1 -> Product1/1
  Constant1/1 -> Product3/1
  Gain2/1 -> Product2/2
  Constant/1 -> Product/2
  Transpose/1 -> Product/1
  Integrator/1 -> Kr/1, Gain/1
  r(t)/1 -> Transpose1/1
  Transpose1/1 -> Product2/1
  Product2/1 -> Sum/2
  Gain/1 -> Sum/1
  saturation/1 -> Product5/2
  saturation_rate/1 -> Product4/2
  Sum/1 -> Product4/1
  Product4/1 -> Product5/1
  Product5/1 -> Integrator/1
  Demux/3 -> Square/1
  e(t)/1 -> Demux/1, Transpose/1
  Square/1 -> Product3/2
  Product3/1 -> Product1/2

== system control_model_5/Subsystem3/phi calculation ==
  x(t) : Inport
  Constant1 : Constant
  Constant2 : Constant  Value=0
  Constant3 : Constant
  Demux1 : Demux
  Divide : Product  Inputs=/*
  Mux2 : Mux  Inputs=5
  Product : Product
  Square : Math  Operator=square
  Square1 : Math  Operator=square
  Square2 : Math  Operator=square
  phi(t) : Outport
  wires:
  Demux1/1 -> Product/1, Square2/1
  Mux2/1 -> phi(t)/1
  x(t)/1 -> Demux1/1
  Demux1/2 -> Product/2, Square1/1
  Demux1/3 -> Square/1
  Constant3/1 -> Mux2/1
  Square1/1 -> Mux2/3
  Square2/1 -> Mux2/2
  Product/1 -> Mux2/4
  Divide/1 -> Mux2/5
  Square/1 -> Divide/1
  Constant1/1 -> Divide/2

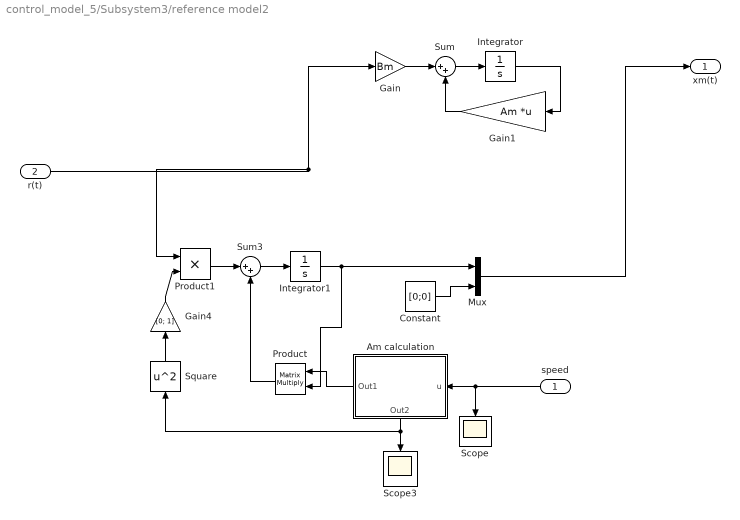
== system control_model_5/Subsystem3/reference model2 ==
  speed : Inport
  r(t) : Inport  Port=2
  Am calculation : Subsystem
      settings: PortSchema="{\"entries\":[{\"content\":{\"sides\":[{\"content\":{\"connectorIds\":[\"In1\"]},\"type\":\"ConnectorPlacement.EquallySpacedRectSide\",\"uuid\":\"0f416610-6d09-41b2-8e43-ab12bae17171\"},{\"content\":{\"connectorIds\":[\"Out1\"],\"side\":\"RIGHT\"},\"type\":\"ConnectorPlacement.EquallySpacedRectSide\",\"uuid\":\"5b01f4e2-a9d9-401f-a995-209f65c9ed0a\"},{\"content\":{\"side\":\"TOP\"},\"type\":\"ConnectorPlacement.EquallySpacedRectSide\",\"uuid\":\"7b4b3b15-4017-4e41-9ba8-195eebb27a5a\"},{\"content\":{\"connectorIds\":[\"Out2\"],\"side\":\"BOTTOM\"},\"type\":\"ConnectorPlacement.EquallySpacedRectSide\",\"uuid\":\"9545ecff-be55-4474-a592-91f309f09551\"}]},\"type\":\"ConnectorPlacement.EquallySpacedConnector\",\"uuid\":\"30f52be7-dacd-4360-890f-cc1c8790a2b3\"}],\"packageUris\":[\"http://schema.mathworks.com/mf0/Connector/R2020b\"],\"version\":\"1.0\"}"
  Constant : Constant  Value=[0;0]
  Gain : Gain  Gain=Bm
  Gain1 : Gain  Gain=Am  Multiplication=Matrix(K*u) (u vector)
  Gain4 : Gain  Gain=[0; 1]
  Integrator : Integrator
  Integrator1 : Integrator  InitialCondition=[0; 0]
  Mux : Mux  Inputs=2
  Product : Product  Multiplication=Matrix(*)
  Product1 : Product
  Scope : Scope
      settings: ActiveDisplayYMinimum=-1  ActiveDisplayYMaximum=1  DataLoggingVariableName=ScopeData27
  Scope3 : Scope
      settings: ActiveDisplayYMinimum=-1  ActiveDisplayYMaximum=1  DataLoggingVariableName=ScopeData30
  Square : Math  Operator=square
  Sum : Sum  Inputs=|++
  Sum3 : Sum  Inputs=|++
  xm(t) : Outport  PortDimensions=[4 1]
  wires:
  Gain/1 -> Sum/1
  Sum/1 -> Integrator/1
  Gain1/1 -> Sum/2
  Integrator/1 -> Gain1/1
  r(t)/1 -> Gain/1, Product1/1
  Integrator1/1 -> Mux/1, Product/2
  Sum3/1 -> Integrator1/1
  Product1/1 -> Sum3/1
  Product/1 -> Sum3/2
  speed/1 -> Scope/1, Am calculation/1(u)
  Am calculation/1(Out1) -> Product/1
  Am calculation/2(Out2) -> Square/1, Scope3/1
  Gain4/1 -> Product1/2
  Square/1 -> Gain4/1
  Constant/1 -> Mux/2
  Mux/1 -> xm(t)/1

== system control_model_5/Subsystem5/Cm_Alpha_calculation ==
  alpha : Inport
  Constant : Constant
  Constant1 : Constant
  Divide : Product  Inputs=*/
  Gain : Gain  Gain=1/deg2rad(15)
  Gain7 : Gain  Gain=Cm_0
  Product : Product
  Scope5 : Scope
      settings: ActiveDisplayYMinimum=-1  ActiveDisplayYMaximum=1  DataLoggingVariableName=ScopeData11
  Square : Math  Operator=square
  Sum : Sum  Inputs=|++
  Cm_alpha : Outport
  wires:
  Product/1 -> Cm_alpha/1
  Gain7/1 -> Scope5/1, Product/2
  Gain/1 -> Square/1
  alpha/1 -> Gain/1, Product/1
  Square/1 -> Sum/1
  Constant/1 -> Sum/2
  Sum/1 -> Divide/2
  Divide/1 -> Gain7/1
  Constant1/1 -> Divide/1

== system control_model_5/Subsystem5/Cm_delta_calculation ==
  AOA : Inport
  Constant11 : Constant  Value=Cm_delta
  Constant2 : Constant
  Divide : Product  Inputs=/*
  Gain5 : Gain  Gain=rate_of_change
  Square : Math  Operator=square
  Sum4 : Sum  Inputs=++|
  Out1 : Outport
  wires:
  Gain5/1 -> Sum4/2
  Constant2/1 -> Sum4/1
  Divide/1 -> Out1/1
  Sum4/1 -> Divide/1
  Constant11/1 -> Divide/2
  Square/1 -> Gain5/1
  AOA/1 -> Square/1

== system control_model_5/Subsystem5/Drag calculations ==
  speed : Inport
  In1 : Inport  Port=2
  AOA : Inport  Port=3
  Constant3 : Constant  Value=Cd0
  Gain5 : Gain  Gain=k_d2
  Gain6 : Gain  Gain=k_d1
  Gain7 : Gain  Gain=S*1/2*rho
  Product : Product
  Square : Math  Operator=square
  Square1 : Math  Operator=square
  Square2 : Math  Operator=square
  Sum3 : Sum  Inputs=+++
  Drag : Outport
  wires:
  Square1/1 -> Gain6/1
  Square2/1 -> Gain5/1
  Product/1 -> Drag/1
  Sum3/1 -> Gain7/1
  Gain6/1 -> Sum3/3
  Gain7/1 -> Product/2
  Constant3/1 -> Sum3/1
  Square/1 -> Product/1
  Gain5/1 -> Sum3/2
  AOA/1 -> Square2/1
  In1/1 -> Square1/1
  speed/1 -> Square/1

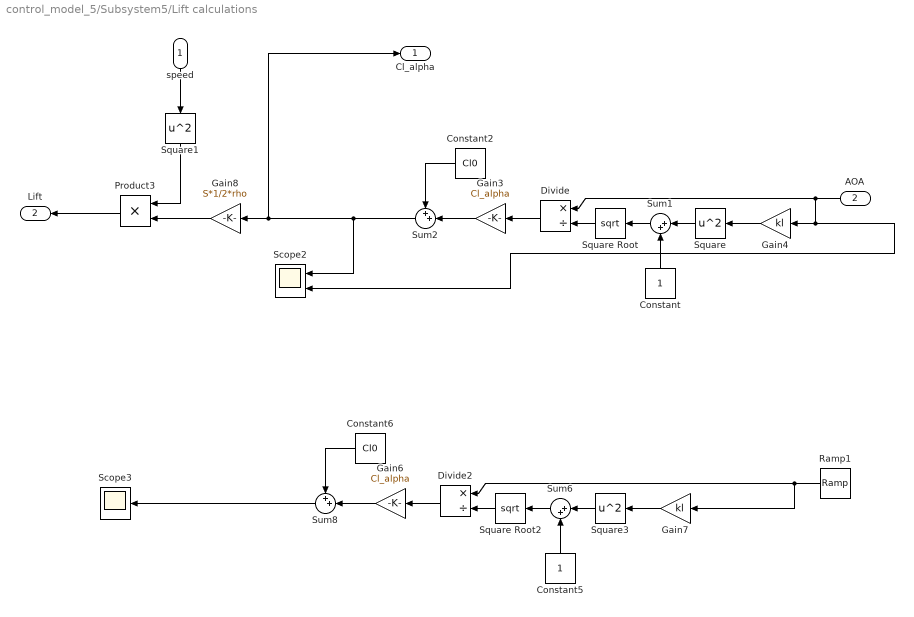
== system control_model_5/Subsystem5/Lift calculations ==
  speed : Inport
  AOA : Inport  Port=2
  Constant : Constant
  Constant2 : Constant  Value=Cl0
  Constant5 : Constant
  Constant6 : Constant  Value=Cl0
  Divide : Product  Inputs=*/
  Divide2 : Product  Inputs=*/
  Gain3 : Gain  Gain=Cl_alpha
  Gain4 : Gain  Gain=kl
  Gain6 : Gain  Gain=Cl_alpha
  Gain7 : Gain  Gain=kl
  Gain8 : Gain  Gain=S*1/2*rho
  Product3 : Product
  Ramp1 : simulink/Sources/Ramp  slope=deg2rad(1)  start=0  InitialOutput=-deg2rad(60)
  Scope2 : Scope  NumInputPorts=2
      settings: ActiveDisplayYMinimum=-3.0358993033761661  ActiveDisplayYMaximum=1.5205805122741798  DataLoggingVariableName=ScopeData9
  Scope3 : Scope
      settings: ActiveDisplayYMinimum=-2.1631149707231323  ActiveDisplayYMaximum=2.3631149707231325  DataLoggingVariableName=ScopeData23
  Square : Math  Operator=square
  Square Root : Sqrt
  Square Root2 : Sqrt
  Square1 : Math  Operator=square
  Square3 : Math  Operator=square
  Sum1 : Sum  Inputs=|++
  Sum2 : Sum  Inputs=++|
  Sum6 : Sum  Inputs=|++
  Sum8 : Sum  Inputs=++|
  Cl_alpha : Outport
  Lift : Outport  Port=2
  wires:
  Square/1 -> Sum1/1
  Square Root/1 -> Divide/2
  Gain3/1 -> Sum2/2
  Constant2/1 -> Sum2/1
  AOA/1 -> Divide/1, Scope2/2, Gain4/1
  Gain4/1 -> Square/1
  Gain8/1 -> Product3/2
  Constant/1 -> Sum1/2
  Divide/1 -> Gain3/1
  Product3/1 -> Lift/1
  Sum1/1 -> Square Root/1
  Square1/1 -> Product3/1
  speed/1 -> Square1/1
  Sum2/1 -> Cl_alpha/1, Gain8/1, Scope2/1
  Square3/1 -> Sum6/1
  Ramp1/1 -> Divide2/1, Gain7/1
  Gain7/1 -> Square3/1
  Gain6/1 -> Sum8/2
  Sum6/1 -> Square Root2/1
  Divide2/1 -> Gain6/1
  Constant6/1 -> Sum8/1
  Constant5/1 -> Sum6/2
  Square Root2/1 -> Divide2/2
  Sum8/1 -> Scope3/1

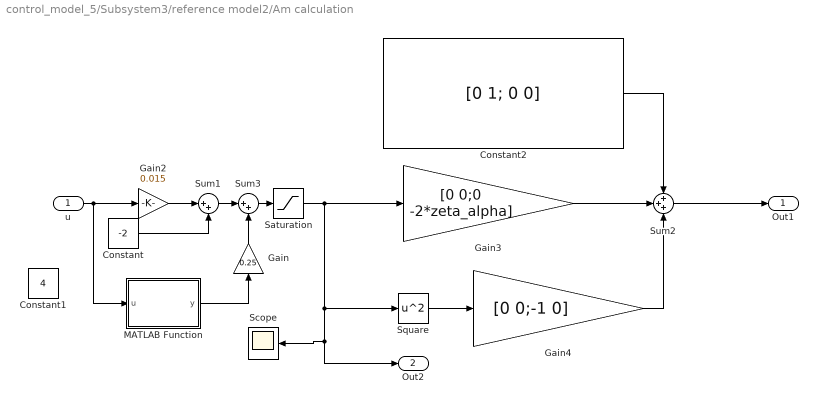
== system control_model_5/Subsystem3/reference model2/Am calculation ==
  u : Inport
  Constant : Constant  Value=-2
  Constant1 : Constant  Value=4
  Constant2 : Constant  Value=[0 1; 0 0]  VectorParams1D=off
  Gain : Gain  Gain=0.25
  Gain2 : Gain  Gain=0.015
  Gain3 : Gain  Gain=[0 0;0 -2*zeta_alpha]
  Gain4 : Gain  Gain=[0 0;-1 0]
  MATLAB Function : MATLAB Function  TreatAsAtomicUnit=on
  Saturation : Saturate  UpperLimit=10  LowerLimit=0.1
  Scope : Scope
      settings: ActiveDisplayYMinimum=-1  ActiveDisplayYMaximum=1  DataLoggingVariableName=ScopeData29
  Square : Math  Operator=square
  Sum1 : Sum  Inputs=|++
  Sum2 : Sum  Inputs=+++
  Sum3 : Sum  Inputs=|++
  Out1 : Outport
  Out2 : Outport  Port=2
  wires:
  Gain4/1 -> Sum2/3
  Constant2/1 -> Sum2/1
  Constant/1 -> Sum1/2
  Square/1 -> Gain4/1
  Gain3/1 -> Sum2/2
  Gain2/1 -> Sum1/1
  Sum2/1 -> Out1/1
  u/1 -> MATLAB Function/1(u), Gain2/1
  Saturation/1 -> Scope/1, Out2/1, Square/1, Gain3/1
  Sum1/1 -> Sum3/1
  Sum3/1 -> Saturation/1
  MATLAB Function/1(y) -> Gain/1
  Gain/1 -> Sum3/2

== matlab function control_model_5/Subsystem3/reference model2/Am calculation/MATLAB Function ==
  data: u input; y output
function y = fcn(u)
if u<200
    y=1;
else
    y=0;
end

== matlab function control_model_5/MATLAB Function2 ==
  data: u input; y output
function y = fcn(u)
if u<33
    y=0;
else
    y=1;
end
